simulink model "HW3_simulink"  (R2019b)
settings: Solver=FixedStepAuto  StartTime=0.0  StopTime=6  RelTol=1e-3
values from neighbouring files (symbols this model uses):
  Aeval = eval(subs(A, {u, v, w, p, q, r, phi, theta, psi, XNED, YNED, ZNED, n1, n2, n3, n4},               {0, 0, 0, 0, 0, 0, 0, 0, 0, 0, 0, 0, 299, 299, 299, 299}))    [HW3.m]
  Beval = eval(subs(B, {u, v, w, p, q, r, phi, theta, psi, XNED, YNED, ZNED, n1, n2, n3, n4},                   {0, 0, 0, 0, 0, 0, 0, 0, 0, 0, 0, 0, 299, 299, 299, 299}))    [HW3.m]
  Ceval = eval(subs(C, {u, v, w, p, q, r, phi, theta, psi, XNED, YNED, ZNED, n1, n2, n3, n4},                   {0, 0, 0, 0, 0, 0, 0, 0, 0, 0, 0, 0, 299, 299, 299, 299}))    [HW3.m]
  Deval = eval(subs(D, {u, v, w, p, q, r, phi, theta, psi, XNED, YNED, ZNED, n1, n2, n3, n4},               {0, 0, 0, 0, 0, 0, 0, 0, 0, 0, 0, 0, 299, 299, 299, 299}))    [HW3.m]
  M_motor = [1, 1, 1, -1;             1, 1, -1, 1;             1, -1, -1, -1;             1, -1, 1, 1 ]    [HW3.m]
settings Model: Creator=whipper  LastModifiedBy=cwhipp

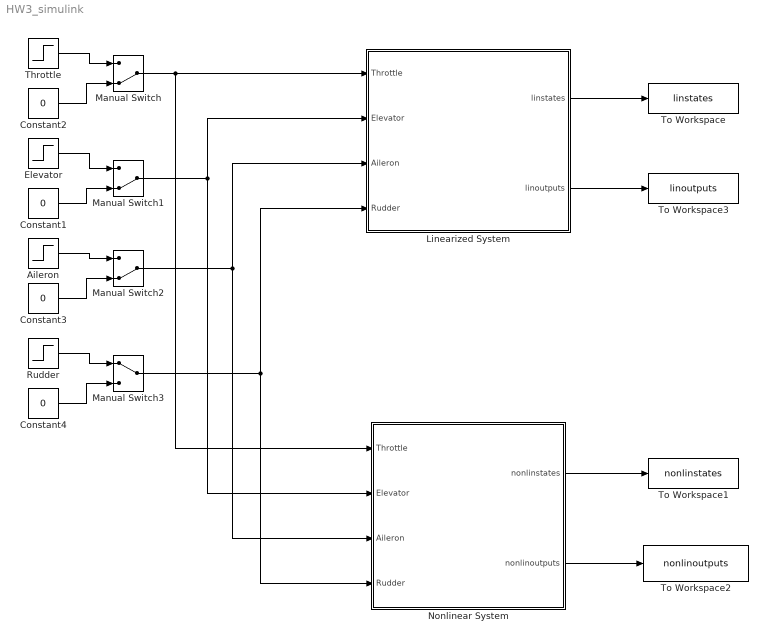
== system HW3_simulink ==
  Aileron : Step  SampleTime=0
  Constant{1..4} (4 alike) : Constant  Value=0
  Elevator : Step  SampleTime=0
  Linearized System : Subsystem
  Manual Switch : ManualSwitch  CurrentSetting=0
  Manual Switch1 : ManualSwitch  CurrentSetting=0
  Manual Switch2 : ManualSwitch  CurrentSetting=0
  Manual Switch3 : ManualSwitch
  Nonlinear System : Subsystem
  Rudder : Step  SampleTime=0
  Throttle : Step  SampleTime=0
  To Workspace : ToWorkspace  VariableName=linstates  SaveFormat=Timeseries  SampleTime=-1
  To Workspace1 : ToWorkspace  VariableName=nonlinstates  SaveFormat=Timeseries  SampleTime=-1
  To Workspace2 : ToWorkspace  VariableName=nonlinoutputs  SaveFormat=Timeseries  SampleTime=-1
  To Workspace3 : ToWorkspace  VariableName=linoutputs  SaveFormat=Timeseries  SampleTime=-1
  wires:
  Constant2/1 -> Manual Switch/2
  Manual Switch/1 -> Nonlinear System/1("Throttle "), Linearized System/1(Throttle)
  Throttle/1 -> Manual Switch/1
  Manual Switch1/1 -> Linearized System/2(Elevator), Nonlinear System/2(Elevator)
  Linearized System/1(linstates) -> To Workspace/1
  Nonlinear System/1("nonlinstates ") -> To Workspace1/1
  Nonlinear System/2(nonlinoutputs) -> To Workspace2/1
  Linearized System/2("linoutputs ") -> To Workspace3/1
  Constant1/1 -> Manual Switch1/2
  Elevator/1 -> Manual Switch1/1
  Constant3/1 -> Manual Switch2/2
  Aileron/1 -> Manual Switch2/1
  Constant4/1 -> Manual Switch3/2
  Rudder/1 -> Manual Switch3/1
  Manual Switch2/1 -> Linearized System/3(Aileron), Nonlinear System/3(Aileron)
  Manual Switch3/1 -> Linearized System/4(Rudder), Nonlinear System/4(Rudder)

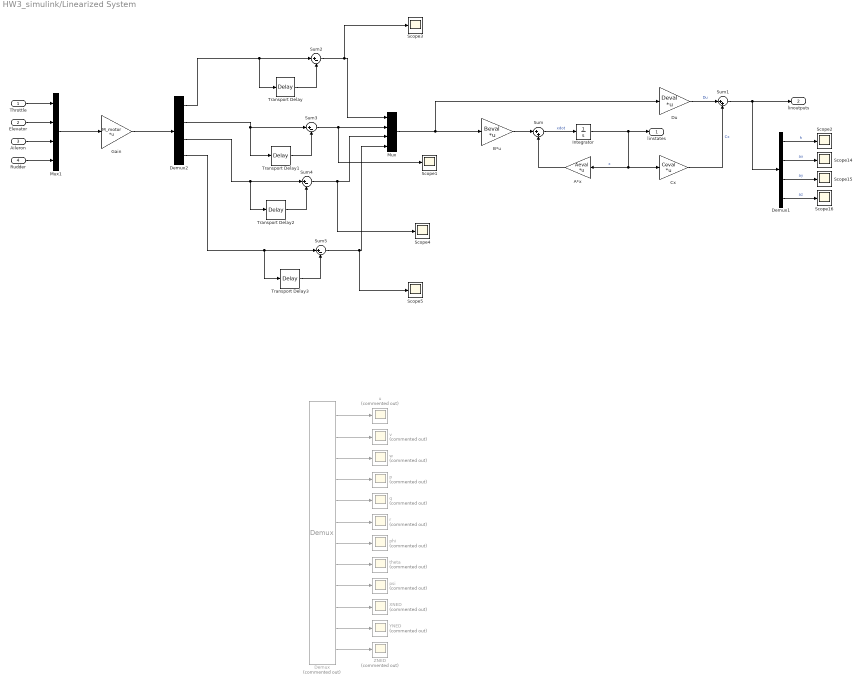
== system HW3_simulink/Linearized System ==
  Throttle : Inport
  Elevator : Inport  Port=2
  Aileron : Inport  Port=3
  Rudder : Inport  Port=4
  A*x : Gain  Gain=Aeval  Multiplication=Matrix(K*u)
  B*u : Gain  Gain=Beval  Multiplication=Matrix(K*u)
  Cx : Gain  Gain=Ceval  Multiplication=Matrix(K*u)
  Demux : Demux  Commented=on  Outputs=12
  Demux1 : Demux
  Demux2 : Demux
  Du : Gain  Gain=Deval  Multiplication=Matrix(K*u)
  Gain : Gain  Gain=M_motor  Multiplication=Matrix(K*u)
  Integrator : Integrator
  Mux : Mux
  Mux1 : Mux
  Scope{1..5,14..16} (8 alike) : Scope
  Sum : Sum  Inputs=|++
  Sum1 : Sum  Inputs=|++
  Sum{2..5} (4 alike) : Sum  Inputs=|+-
  Transport Delay{,1..3} (4 alike) : TransportDelay  DelayTime=4
  XNED : Scope  Commented=on
  YNED : Scope  Commented=on
  ZNED : Scope  Commented=on
  p : Scope  Commented=on
  phi : Scope  Commented=on
  psi : Scope  Commented=on
  q : Scope  Commented=on
  r : Scope  Commented=on
  theta : Scope  Commented=on
  u : Scope  Commented=on
  v : Scope  Commented=on
  w : Scope  Commented=on
  linstates : Outport
  "linoutputs " : Outport  Port=2
  wires:
  Sum/1 -> Integrator/1  "xdot"
  A*x/1 -> Sum/2
  Du/1 -> Sum1/1  "Du"
  Integrator/1 -> Cx/1, A*x/1, linstates/1  "x"
  Sum1/1 -> Demux1/1, "linoutputs "/1
  Mux/1 -> Du/1, B*u/1
  B*u/1 -> Sum/1
  Sum3/1 -> Scope1/1, Mux/2
  Cx/1 -> Sum1/2  "Cx"
  Demux/1 -> u/1
  Demux/2 -> v/1
  Demux/3 -> w/1
  Demux/4 -> p/1
  Demux/5 -> q/1
  Demux/6 -> r/1
  Demux/7 -> phi/1
  Demux/8 -> theta/1
  Demux/9 -> psi/1
  Demux/10 -> XNED/1
  Demux/11 -> YNED/1
  Demux/12 -> ZNED/1
  Demux1/1 -> Scope2/1  "h"
  Demux1/2 -> Scope14/1  "ax"
  Demux1/3 -> Scope15/1  "ay"
  Demux1/4 -> Scope16/1  "az"
  Transport Delay1/1 -> Sum3/2
  Demux2/2 -> Transport Delay1/1, Sum3/1
  Sum2/1 -> Scope3/1, Mux/1
  Demux2/1 -> Transport Delay/1, Sum2/1
  Transport Delay/1 -> Sum2/2
  Sum4/1 -> Scope4/1, Mux/3
  Demux2/3 -> Sum4/1, Transport Delay2/1
  Transport Delay2/1 -> Sum4/2
  Sum5/1 -> Scope5/1, Mux/4
  Demux2/4 -> Sum5/1, Transport Delay3/1
  Transport Delay3/1 -> Sum5/2
  Mux1/1 -> Gain/1
  Gain/1 -> Demux2/1
  Rudder/1 -> Mux1/4
  Aileron/1 -> Mux1/3
  Elevator/1 -> Mux1/2
  Throttle/1 -> Mux1/1

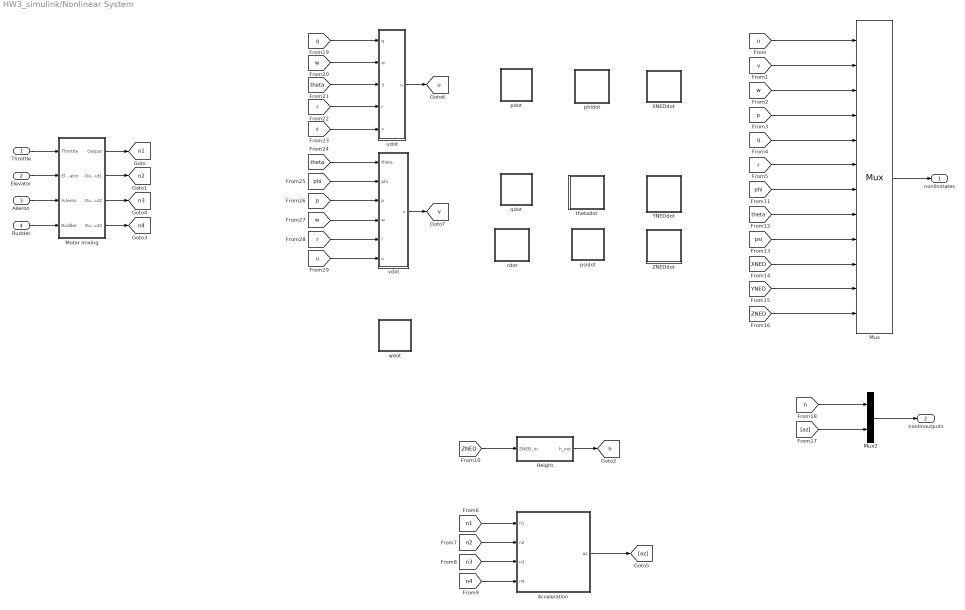
== system HW3_simulink/Nonlinear System ==
  "Throttle " : Inport
  Elevator : Inport  Port=2
  Aileron : Inport  Port=3
  Rudder : Inport  Port=4
  Acceleration : Subsystem
  Height : Subsystem
  "Motor mixing " : Subsystem
  Mux : Mux  Inputs=12
  Mux2 : Mux  Inputs=2
  "XNEDdot " : Subsystem
  "YNEDdot " : Subsystem
  ZNEDdot : Subsystem
  pdot : Subsystem
  phidot : Subsystem
  "psidot " : Subsystem
  qdot : Subsystem
  rdot : Subsystem
  "thetadot " : Subsystem
  udot : Subsystem
  vdot : Subsystem
  "wdot " : Subsystem
  "nonlinstates " : Outport
  nonlinoutputs : Outport  Port=2
  tag scope: h=global, n1=global, n2=global, n3=global, n4=global, u=global, v=global
  wires:
  [n2] -> Acceleration/2(n2)
  [n1] -> Acceleration/1(n1)
  [n3] -> Acceleration/3(n3)
  Acceleration/1(az) -> [az]
  [n4] -> Acceleration/4(n4)
  [ZNED] -> Height/1("ZNED_in ")
  Height/1("h_out ") -> [h]
  [phi] -> Mux/7
  [theta] -> Mux/8
  [psi] -> Mux/9
  [XNED] -> Mux/10
  [YNED] -> Mux/11
  [ZNED] -> Mux/12
  [u] -> Mux/1
  [v] -> Mux/2
  [w] -> Mux/3
  [p] -> Mux/4
  [q] -> Mux/5
  [r] -> Mux/6
  Mux/1 -> "nonlinstates "/1
  [h] -> Mux2/1
  [az] -> Mux2/2
  Mux2/1 -> nonlinoutputs/1
  udot/1("u ") -> [u]
  [q] -> udot/1("q ")
  [w] -> udot/2("w ")
  [theta] -> udot/3(theta)
  [r] -> udot/4("r ")
  [v] -> udot/5(v)
  "Throttle "/1 -> "Motor mixing "/1("Throttle ")
  Elevator/1 -> "Motor mixing "/2(Elevator)
  Aileron/1 -> "Motor mixing "/3(Aileron)
  Rudder/1 -> "Motor mixing "/4(Rudder)
  "Motor mixing "/1(Output) -> [n1]
  "Motor mixing "/2(Output1) -> [n2]
  "Motor mixing "/3(Output2) -> [n3]
  "Motor mixing "/4(Output3) -> [n4]
  [theta] -> vdot/1(theta)
  [phi] -> vdot/2(phi)
  [p] -> vdot/3(p)
  [w] -> vdot/4(w)
  [r] -> vdot/5(r)
  [u] -> vdot/6(u)
  vdot/1(v) -> [v]

== system HW3_simulink/Nonlinear System/Acceleration ==
  n1 : Inport
  n2 : Inport  Port=2
  n3 : Inport  Port=3
  n4 : Inport  Port=4
  Gain : Gain  Gain=1.9060e-06
  Square{,1..3} (4 alike) : Math  Operator=square  SignedPower=off  SaturateOnIntegerOverflow=on
  Sum : Sum  Inputs=----
  az : Outport
  wires:
  n1/1 -> Square/1
  n2/1 -> Square1/1
  n3/1 -> Square2/1
  n4/1 -> Square3/1
  Square/1 -> Sum/1
  Square1/1 -> Sum/2
  Square2/1 -> Sum/3
  Square3/1 -> Sum/4
  Sum/1 -> Gain/1
  Gain/1 -> az/1

== system HW3_simulink/Nonlinear System/Height ==
  "ZNED_in " : Inport
  Gain : Gain  Gain=-1
  "h_out " : Outport
  wires:
  "ZNED_in "/1 -> Gain/1
  Gain/1 -> "h_out "/1

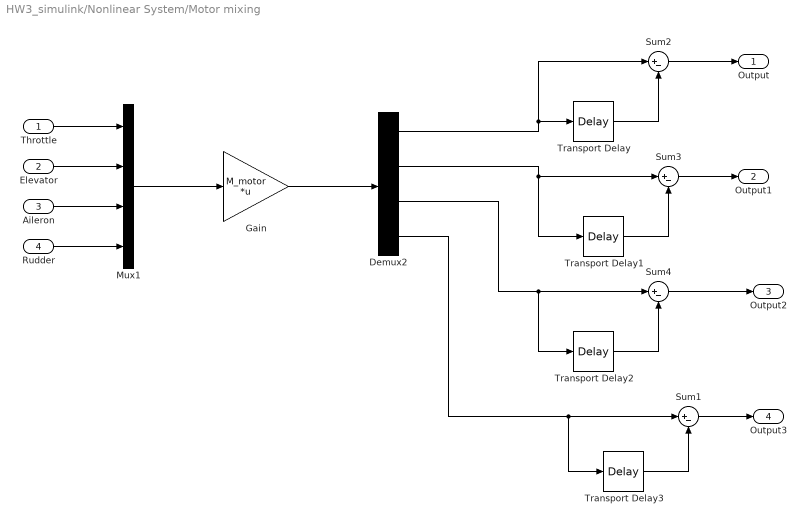
== system HW3_simulink/Nonlinear System/Motor mixing  ==
  "Throttle " : Inport
  Elevator : Inport  Port=2
  Aileron : Inport  Port=3
  Rudder : Inport  Port=4
  Demux2 : Demux
  Gain : Gain  Gain=M_motor  Multiplication=Matrix(K*u)
  Mux1 : Mux
  Sum{1..4} (4 alike) : Sum  Inputs=|+-
  Transport Delay{,1..3} (4 alike) : TransportDelay  DelayTime=4
  Output : Outport
  Output1 : Outport  Port=2
  Output2 : Outport  Port=3
  Output3 : Outport  Port=4
  wires:
  Rudder/1 -> Mux1/4
  Transport Delay2/1 -> Sum4/2
  "Throttle "/1 -> Mux1/1
  Transport Delay3/1 -> Sum1/2
  Sum4/1 -> Output2/1
  Sum3/1 -> Output1/1
  Sum2/1 -> Output/1
  Transport Delay/1 -> Sum2/2
  Aileron/1 -> Mux1/3
  Gain/1 -> Demux2/1
  Demux2/2 -> Transport Delay1/1, Sum3/1
  Transport Delay1/1 -> Sum3/2
  Demux2/3 -> Sum4/1, Transport Delay2/1
  Sum1/1 -> Output3/1
  Demux2/1 -> Sum2/1, Transport Delay/1
  Mux1/1 -> Gain/1
  Elevator/1 -> Mux1/2
  Demux2/4 -> Transport Delay3/1, Sum1/1

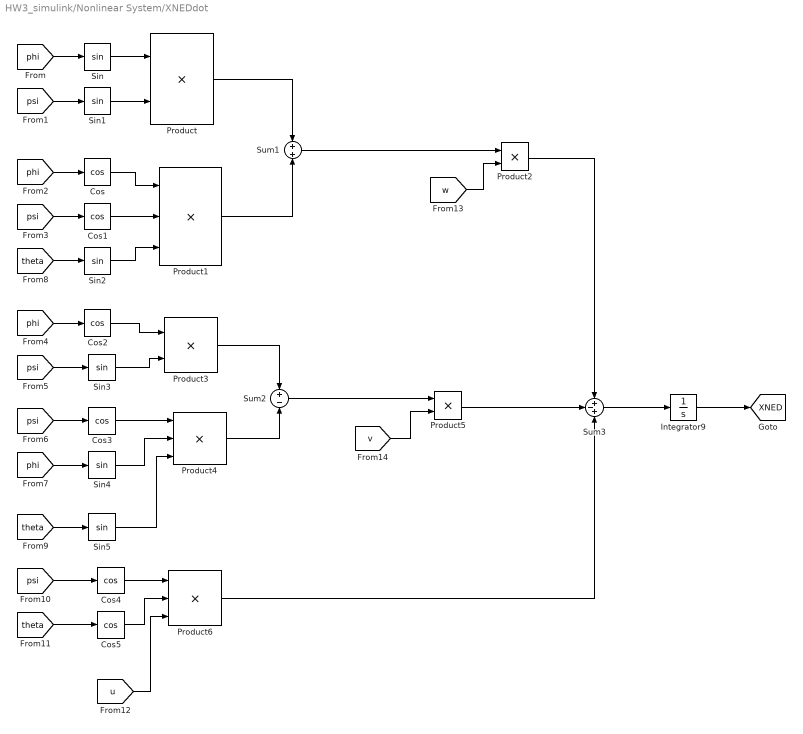
== system HW3_simulink/Nonlinear System/XNEDdot  ==
  Cos{,1..5} (6 alike) : Trigonometry  Operator=cos
  Integrator9 : Integrator
  Product{,2..3,5} (4 alike) : Product
  Product1 : Product  Inputs=3
  Product4 : Product  Inputs=3
  Product6 : Product  Inputs=3
  Sin{,1..5} (6 alike) : Trigonometry
  Sum1 : Sum
  Sum2 : Sum  Inputs=+-
  Sum3 : Sum  Inputs=+-+
  tag scope: XNED=global
  wires:
  Cos1/1 -> Product1/2
  [psi] -> Sin1/1
  Sum1/1 -> Product2/1
  Product1/1 -> Sum1/2
  Product/1 -> Sum1/1
  Sin1/1 -> Product/2
  [phi] -> Sin/1
  Sin/1 -> Product/1
  Cos/1 -> Product1/1
  [theta] -> Sin2/1
  Sin2/1 -> Product1/3
  [w] -> Product2/2
  Product4/1 -> Sum2/2
  [v] -> Product5/2
  Product3/1 -> Sum2/1
  Sum2/1 -> Product5/1
  Cos5/1 -> Product6/2
  [u] -> Product6/3
  Product2/1 -> Sum3/1
  Product5/1 -> Sum3/2
  Product6/1 -> Sum3/3
  Sum3/1 -> Integrator9/1
  Integrator9/1 -> [XNED]
  [phi] -> Cos/1
  [psi] -> Cos1/1
  [phi] -> Cos2/1
  Cos2/1 -> Product3/1
  [psi] -> Sin3/1
  Sin3/1 -> Product3/2
  [psi] -> Cos3/1
  Cos3/1 -> Product4/1
  [phi] -> Sin4/1
  Sin4/1 -> Product4/2
  [theta] -> Sin5/1
  Sin5/1 -> Product4/3
  [psi] -> Cos4/1
  Cos4/1 -> Product6/1
  [theta] -> Cos5/1

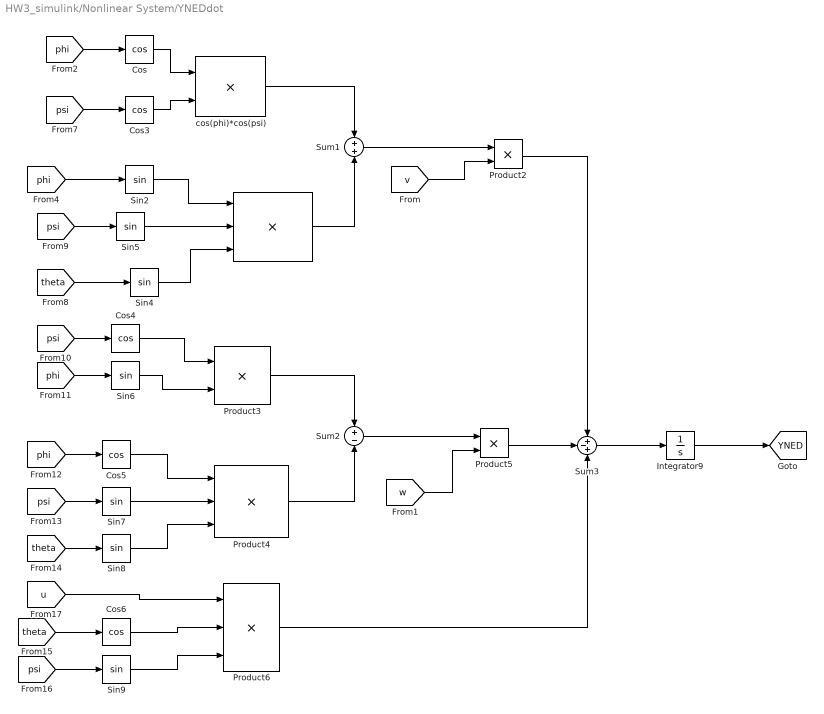
== system HW3_simulink/Nonlinear System/YNEDdot  ==
  " " : Product  Inputs=3
  Cos{,3..6} (5 alike) : Trigonometry  Operator=cos
  Integrator9 : Integrator
  Product2 : Product
  Product3 : Product
  Product4 : Product  Inputs=3
  Product5 : Product
  Product6 : Product  Inputs=3
  Sin{2,4..9} (7 alike) : Trigonometry
  Sum1 : Sum
  Sum2 : Sum  Inputs=+-
  Sum3 : Sum  Inputs=+-+
  cos(phi)*cos(psi) : Product
  tag scope: YNED=global
  wires:
  Product3/1 -> Sum2/1
  Product2/1 -> Sum3/1
  cos(phi)*cos(psi)/1 -> Sum1/1
  Sum1/1 -> Product2/1
  Integrator9/1 -> [YNED]
  [v] -> Product2/2
  Sum3/1 -> Integrator9/1
  Sum2/1 -> Product5/1
  " "/1 -> Sum1/2
  Product6/1 -> Sum3/3
  [w] -> Product5/2
  Product4/1 -> Sum2/2
  Product5/1 -> Sum3/2
  Cos/1 -> cos(phi)*cos(psi)/1
  [phi] -> Cos/1
  [phi] -> Sin2/1
  Sin2/1 -> " "/1
  [psi] -> Cos3/1
  Cos3/1 -> cos(phi)*cos(psi)/2
  Sin5/1 -> " "/2
  [psi] -> Sin5/1
  [psi] -> Cos4/1
  Cos4/1 -> Product3/1
  [phi] -> Sin6/1
  Sin6/1 -> Product3/2
  [phi] -> Cos5/1
  Cos5/1 -> Product4/1
  [psi] -> Sin7/1
  Sin7/1 -> Product4/2
  [theta] -> Sin8/1
  Sin8/1 -> Product4/3
  [theta] -> Cos6/1
  [psi] -> Sin9/1
  [theta] -> Sin4/1
  Sin4/1 -> " "/3
  [u] -> Product6/1
  Cos6/1 -> Product6/2
  Sin9/1 -> Product6/3

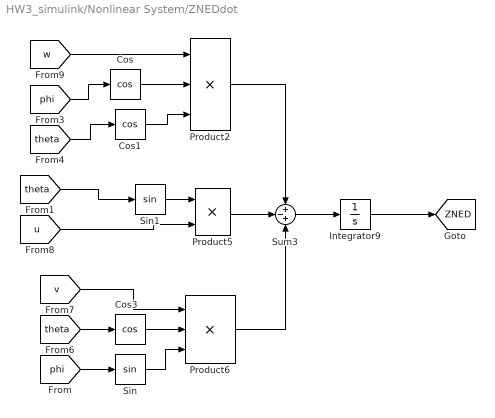
== system HW3_simulink/Nonlinear System/ZNEDdot ==
  Cos : Trigonometry  Operator=cos
  Cos1 : Trigonometry  Operator=cos
  Cos3 : Trigonometry  Operator=cos
  Integrator9 : Integrator
  Product2 : Product  Inputs=3
  Product5 : Product
  Product6 : Product  Inputs=3
  Sin : Trigonometry
  Sin1 : Trigonometry
  Sum3 : Sum  Inputs=+-+
  tag scope: ZNED=global
  wires:
  Product6/1 -> Sum3/3
  [phi] -> Sin/1
  Sum3/1 -> Integrator9/1
  Product2/1 -> Sum3/1
  Product5/1 -> Sum3/2
  [u] -> Product5/2
  Integrator9/1 -> [ZNED]
  [theta] -> Sin1/1
  Cos/1 -> Product2/2
  Cos1/1 -> Product2/3
  Sin1/1 -> Product5/1
  [phi] -> Cos/1
  [theta] -> Cos1/1
  [theta] -> Cos3/1
  [w] -> Product2/1
  Cos3/1 -> Product6/2
  Sin/1 -> Product6/3
  [v] -> Product6/1

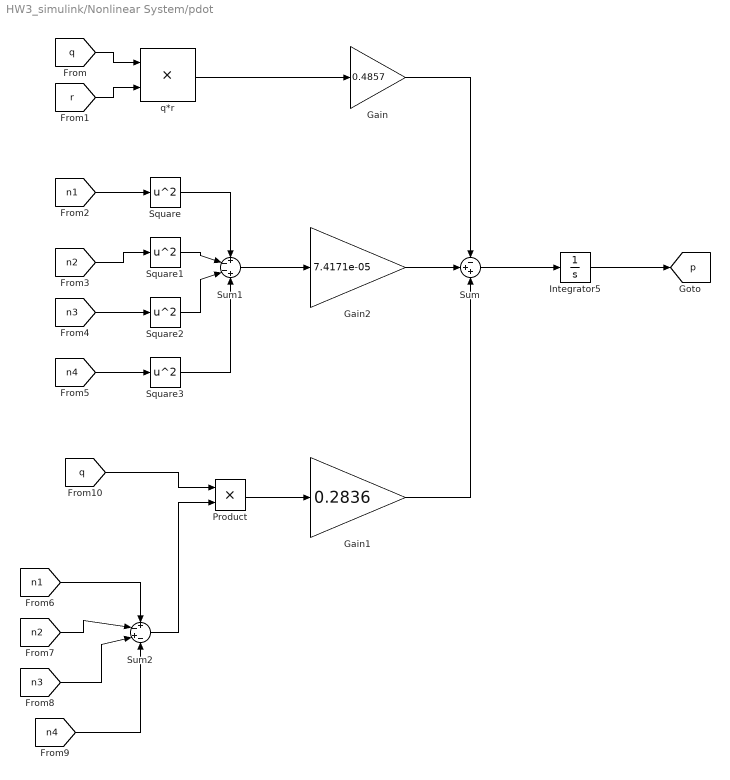
== system HW3_simulink/Nonlinear System/pdot ==
  Gain : Gain  Gain=0.4857
  Gain1 : Gain  Gain=0.2836
  Gain2 : Gain  Gain=7.4171e-05
  Integrator5 : Integrator
  Product : Product
  Square{,1..3} (4 alike) : Math  Operator=square  SignedPower=off  SaturateOnIntegerOverflow=on
  Sum : Sum  Inputs=-++
  Sum1 : Sum  Inputs=+--+
  Sum2 : Sum  Inputs=+-+-
  q*r : Product
  tag scope: p=global
  wires:
  Square1/1 -> Sum1/2
  Sum/1 -> Integrator5/1
  Square2/1 -> Sum1/3
  Square/1 -> Sum1/1
  Integrator5/1 -> [p]
  Square3/1 -> Sum1/4
  [n3] -> Square2/1
  [n1] -> Square/1
  [n4] -> Square3/1
  [n2] -> Square1/1
  [r] -> q*r/2
  [q] -> q*r/1
  q*r/1 -> Gain/1
  Sum1/1 -> Gain2/1
  Sum2/1 -> Product/2
  Product/1 -> Gain1/1
  Gain1/1 -> Sum/3
  [n1] -> Sum2/1
  [n4] -> Sum2/4
  [n3] -> Sum2/3
  [n2] -> Sum2/2
  [q] -> Product/1
  Gain/1 -> Sum/1
  Gain2/1 -> Sum/2

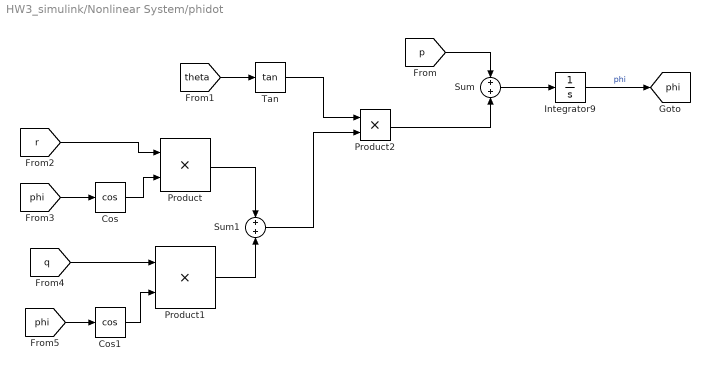
== system HW3_simulink/Nonlinear System/phidot ==
  Cos : Trigonometry  Operator=cos
  Cos1 : Trigonometry  Operator=cos
  Integrator9 : Integrator
  Product : Product
  Product1 : Product
  Product2 : Product
  Sum : Sum
  Sum1 : Sum
  Tan : Trigonometry  Operator=tan
  tag scope: phi=global
  wires:
  Integrator9/1 -> [phi]  "phi"
  [theta] -> Tan/1
  [phi] -> Cos/1
  [p] -> Sum/1
  [q] -> Product1/1
  [r] -> Product/1
  Cos/1 -> Product/2
  Product/1 -> Sum1/1
  Product1/1 -> Sum1/2
  Tan/1 -> Product2/1
  Sum1/1 -> Product2/2
  Product2/1 -> Sum/2
  Sum/1 -> Integrator9/1
  Cos1/1 -> Product1/2
  [phi] -> Cos1/1

== system HW3_simulink/Nonlinear System/psidot  ==
  1/cos(theta) : Fcn  Expr=1/cos(u)
  Cos : Trigonometry  Operator=cos
  Integrator9 : Integrator
  Product : Product
  Product1 : Product
  Product2 : Product
  Sin : Trigonometry
  Sum1 : Sum
  tag scope: psi=global
  wires:
  [q] -> Product1/1
  Cos/1 -> Product/2
  Product1/1 -> Sum1/2
  Integrator9/1 -> [psi]
  Sin/1 -> Product1/2
  Product/1 -> Sum1/1
  [r] -> Product/1
  [phi] -> Cos/1
  Sum1/1 -> Product2/1
  [theta] -> 1/cos(theta)/1
  1/cos(theta)/1 -> Product2/2
  Product2/1 -> Integrator9/1
  [phi] -> Sin/1

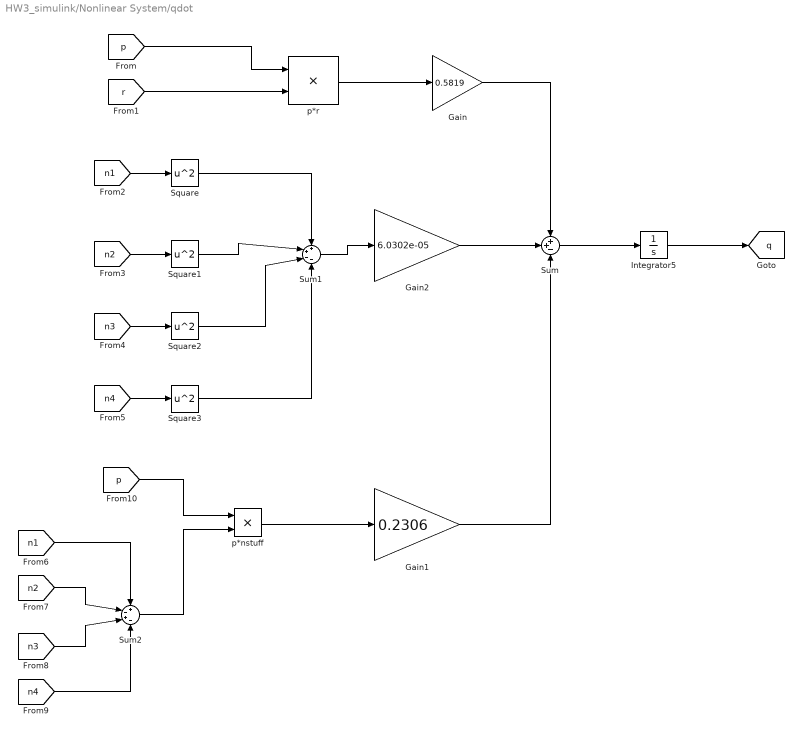
== system HW3_simulink/Nonlinear System/qdot ==
  Gain : Gain  Gain=0.5819
  Gain1 : Gain  Gain=0.2306
  Gain2 : Gain  Gain=6.0302e-05
  Integrator5 : Integrator
  Square{,1..3} (4 alike) : Math  Operator=square  SignedPower=off  SaturateOnIntegerOverflow=on
  Sum : Sum  Inputs=++-
  Sum1 : Sum  Inputs=++--
  Sum2 : Sum  Inputs=+-+-
  p*nstuff : Product
  p*r : Product
  tag scope: q=global
  wires:
  [p] -> p*r/1
  Sum/1 -> Integrator5/1
  Gain1/1 -> Sum/3
  [n2] -> Square1/1
  [r] -> p*r/2
  Square3/1 -> Sum1/4
  Square1/1 -> Sum1/2
  p*nstuff/1 -> Gain1/1
  Integrator5/1 -> [q]
  p*r/1 -> Gain/1
  Square/1 -> Sum1/1
  Sum1/1 -> Gain2/1
  [n3] -> Square2/1
  Square2/1 -> Sum1/3
  [n4] -> Square3/1
  [n1] -> Square/1
  Sum2/1 -> p*nstuff/2
  Gain2/1 -> Sum/2
  Gain/1 -> Sum/1
  [n4] -> Sum2/4
  [n2] -> Sum2/2
  [n3] -> Sum2/3
  [n1] -> Sum2/1
  [p] -> p*nstuff/1

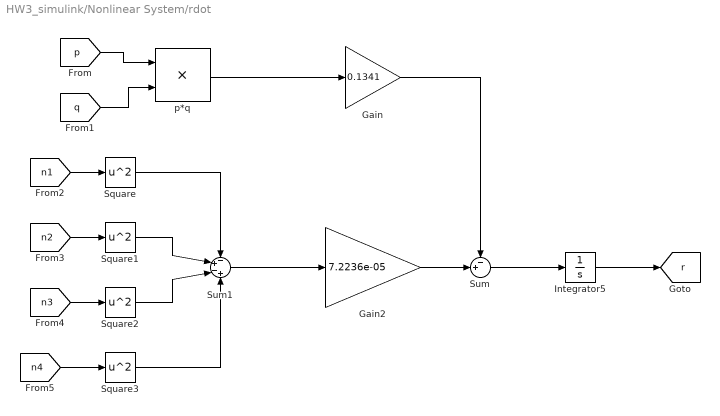
== system HW3_simulink/Nonlinear System/rdot ==
  Gain : Gain  Gain=0.1341
  Gain2 : Gain  Gain=7.2236e-05
  Integrator5 : Integrator
  Square{,1..3} (4 alike) : Math  Operator=square  SignedPower=off  SaturateOnIntegerOverflow=on
  Sum : Sum  Inputs=-+|
  Sum1 : Sum  Inputs=-+-+
  p*q : Product
  tag scope: r=global
  wires:
  [n3] -> Square2/1
  Gain/1 -> Sum/1
  [n4] -> Square3/1
  [q] -> p*q/2
  Square/1 -> Sum1/1
  p*q/1 -> Gain/1
  Square1/1 -> Sum1/2
  Sum/1 -> Integrator5/1
  [p] -> p*q/1
  [n2] -> Square1/1
  [n1] -> Square/1
  Sum1/1 -> Gain2/1
  Square2/1 -> Sum1/3
  Square3/1 -> Sum1/4
  Gain2/1 -> Sum/2
  Integrator5/1 -> [r]

== system HW3_simulink/Nonlinear System/thetadot  ==
  Cos : Trigonometry  Operator=cos
  Integrator9 : Integrator
  Product : Product
  Product1 : Product
  Sin : Trigonometry
  Sum1 : Sum  Inputs=+-
  tag scope: theta=global
  wires:
  [phi] -> Cos/1
  Cos/1 -> Product/2
  [r] -> Product1/1
  Product1/1 -> Sum1/2
  Integrator9/1 -> [theta]  "theta"
  Sin/1 -> Product1/2
  Product/1 -> Sum1/1
  [q] -> Product/1
  Sum1/1 -> Integrator9/1
  [phi] -> Sin/1

== system HW3_simulink/Nonlinear System/udot ==
  "q " : Inport
  "w " : Inport  Port=2
  theta : Inport  Port=3
  "r " : Inport  Port=4
  v : Inport  Port=5
  Gain : Gain  Gain=9.81
  Integrator5 : Integrator
  Sin : Trigonometry
  Sum : Sum  Inputs=+--
  q*w : Product
  r*v : Product
  "u " : Outport
  wires:
  Integrator5/1 -> "u "/1  "u"
  "q "/1 -> q*w/1
  "w "/1 -> q*w/2
  q*w/1 -> Sum/1
  theta/1 -> Sin/1
  Sin/1 -> Gain/1
  Gain/1 -> Sum/2
  "r "/1 -> r*v/1
  v/1 -> r*v/2
  r*v/1 -> Sum/3
  Sum/1 -> Integrator5/1

== system HW3_simulink/Nonlinear System/vdot ==
  theta : Inport
  phi : Inport  Port=2
  p : Inport  Port=3
  w : Inport  Port=4
  r : Inport  Port=5
  u : Inport  Port=6
  Cos : Trigonometry  Operator=cos
  Gain : Gain  Gain=9.81
  Integrator5 : Integrator
  Product : Product
  Sin : Trigonometry
  Sum : Sum  Inputs=+-+
  p*w : Product
  r*u : Product
  v : Outport
  wires:
  r/1 -> r*u/1
  p/1 -> p*w/1
  Sum/1 -> Integrator5/1
  Integrator5/1 -> v/1  "v"
  w/1 -> p*w/2
  u/1 -> r*u/2
  r*u/1 -> Sum/3
  theta/1 -> Cos/1
  Cos/1 -> Product/1
  Sin/1 -> Product/2
  phi/1 -> Sin/1
  Product/1 -> Gain/1
  Gain/1 -> Sum/1
  p*w/1 -> Sum/2

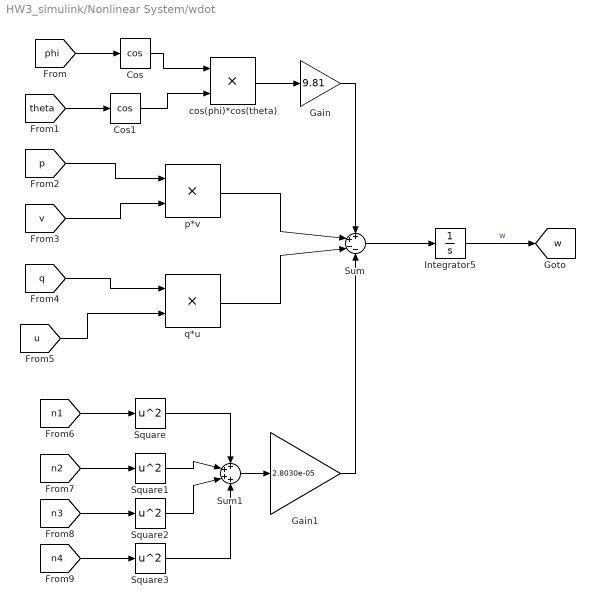
== system HW3_simulink/Nonlinear System/wdot  ==
  Cos : Trigonometry  Operator=cos
  Cos1 : Trigonometry  Operator=cos
  Gain : Gain  Gain=9.81
  Gain1 : Gain  Gain=2.8030e-05
  Integrator5 : Integrator
  Square{,1..3} (4 alike) : Math  Operator=square  SignedPower=off  SaturateOnIntegerOverflow=on
  Sum : Sum  Inputs=++--
  Sum1 : Sum  Inputs=++++
  cos(phi)*cos(theta) : Product
  p*v : Product
  q*u : Product
  tag scope: w=global
  wires:
  q*u/1 -> Sum/3
  [u] -> q*u/2
  Integrator5/1 -> [w]  "w"
  Gain/1 -> Sum/1
  [q] -> q*u/1
  Sum/1 -> Integrator5/1
  [v] -> p*v/2
  [p] -> p*v/1
  p*v/1 -> Sum/2
  [theta] -> Cos1/1
  Cos1/1 -> cos(phi)*cos(theta)/2
  Cos/1 -> cos(phi)*cos(theta)/1
  cos(phi)*cos(theta)/1 -> Gain/1
  [phi] -> Cos/1
  [n1] -> Square/1
  Gain1/1 -> Sum/4
  Square/1 -> Sum1/1
  [n2] -> Square1/1
  [n3] -> Square2/1
  [n4] -> Square3/1
  Square1/1 -> Sum1/2
  Square2/1 -> Sum1/3
  Square3/1 -> Sum1/4
  Sum1/1 -> Gain1/1
